simulink model "imu"  (R2015a)
settings: Solver=FixedStepDiscrete  StartTime=0.0  StopTime=inf  FixedStep=sample_time  RelTol=1e-3
values from neighbouring files (symbols this model uses):
  sample_time = 0.001    [ElmoIncremental.m]    (also in MedullaEncoder.m)
undefined symbols (not defined in the file or in its folder): imu_heading, imu_latitude, imu_reset_cmd
settings Model: xpc_rtwmakecfg_data=_xpcethercatlib_  SimulationMode=external  CovSFcnEnable=off  Creator=wmartin  LastModifiedBy=drl
settings SolverCC: EnableConcurrentExecution=on
settings DataIOCC: MaxDataPoints=1000000000  SaveFormat=StructureWithTime  SaveOutput=off  SaveTime=off
settings OptimizationCC: BlockReduction=off  OptimizeBlockIOStorage=off  BufferReuse=off  GlobalBufferReuse=off  ExpressionFolding=off  ExpressionDepthLimit=2147483647  LocalBlockOutputs=off  SimCompilerOptimization=on
settings DebuggingCC: ArtificialAlgebraicLoopMsg=none  UnderspecifiedInitializationDetection=Classic  MergeDetectMultiDrivingBlocksExec=none  SolverPrmCheckMsg=warning  StateNameClashWarn=warning
settings HardwareCC: ProdIntDivRoundTo=Zero  ProdEndianess=LittleEndian  ProdLongLongMode=on  ProdHWDeviceType=Generic->32-bit x86 compatible
settings ModelReferenceCC: EnableParallelModelReferenceBuilds=on  ModelReferenceNumInstancesAllowed=Single  ModelReferenceMinAlgLoopOccurrences=on
settings RTWCC: SystemTargetFile=slrt.tlc  TemplateMakefile=slrt_default_tmf  Description=Simulink Real-Time  RTWVerbose=off  RTWCompilerOptimization=on
settings CodeAppCC: MaxIdLength=256
settings SimulinkRealTimeCC: GeneratePreprocessorConditionals=Disable all  RL32LogBufSizeModifier=100000000

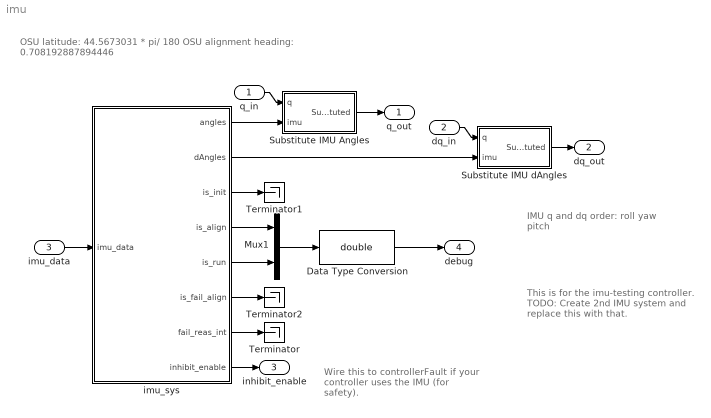
== system imu ==
  note: Wire this to controllerFault
      | if your controller uses the IMU
      | (for safety).
  note: This is for the imu-testing controller.
      | TODO: Create 2nd IMU system and
      | replace this with that.
  note: IMU q and dq order:
      | 	roll
      | 	yaw
      | 	pitch
  note: OSU latitude: 44.5673031 * pi/ 180
      | OSU alignment heading: 0.708192887894446
  q_in : Inport
  dq_in : Inport  Port=2
  imu_data : Inport  Port=3
  Data Type Conversion : DataTypeConversion  OutDataTypeStr=double
  Mux1 : Mux  Inputs=2
  Substitute IMU Angles : Subsystem
  Substitute IMU dAngles : Subsystem
  Terminator : Terminator
  Terminator1 : Terminator
  Terminator2 : Terminator
  imu_sys : MATLAB Function  TreatAsAtomicUnit=on
  q_out : Outport
  dq_out : Outport  Port=2
  inhibit_enable : Outport  Port=3
  debug : Outport  Port=4
  wires:
  imu_data/1 -> imu_sys/1(imu_data)
  imu_sys/1(angles) -> Substitute IMU Angles/2(imu)
  imu_sys/2(dAngles) -> Substitute IMU dAngles/2(imu)
  imu_sys/8(inhibit_enable) -> inhibit_enable/1
  imu_sys/7(fail_reas_int) -> Terminator/1
  imu_sys/6(is_fail_align) -> Terminator2/1
  imu_sys/3(is_init) -> Terminator1/1
  imu_sys/4(is_align) -> Mux1/1
  imu_sys/5(is_run) -> Mux1/2
  Mux1/1 -> Data Type Conversion/1
  Data Type Conversion/1 -> debug/1
  q_in/1 -> Substitute IMU Angles/1(q)
  dq_in/1 -> Substitute IMU dAngles/1(q)
  Substitute IMU Angles/1(Substituted) -> q_out/1
  Substitute IMU dAngles/1(Substituted) -> dq_out/1

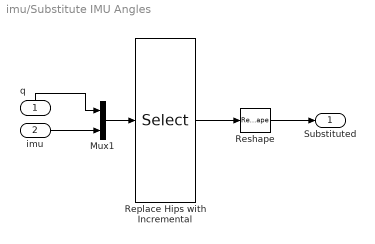
== system imu/Substitute IMU Angles ==
  q : Inport
  imu : Inport  Port=2
  Mux1 : Mux  Inputs=2
  Replace Hips with Incremental : Selector  InputPortWidth=16  Indices=[1 2 3 4 5 6 7 8 9 10 14 15 16]
  Reshape : Reshape
  Substituted : Outport
  wires:
  imu/1 -> Mux1/2
  q/1 -> Mux1/1
  Replace Hips with Incremental/1 -> Reshape/1
  Mux1/1 -> Replace Hips with Incremental/1
  Reshape/1 -> Substituted/1

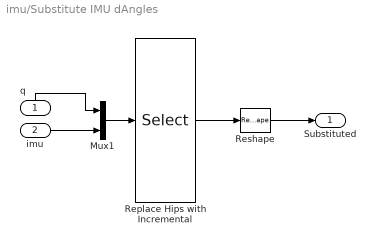
== system imu/Substitute IMU dAngles ==
  q : Inport
  imu : Inport  Port=2
  Mux1 : Mux  Inputs=2
  Replace Hips with Incremental : Selector  InputPortWidth=16  Indices=[1 2 3 4 5 6 7 8 9 10 14 15 16]
  Reshape : Reshape
  Substituted : Outport
  wires:
  Reshape/1 -> Substituted/1
  Mux1/1 -> Replace Hips with Incremental/1
  Replace Hips with Incremental/1 -> Reshape/1
  q/1 -> Mux1/1
  imu/1 -> Mux1/2

== matlab function imu/imu_sys ==
  data: imu_data input size=9; imu_latitude parameter size=1; imu_heading parameter size=1; angles output size=[3 1]; dAngles output size=[3 1]; sample_time parameter size=1; is_init output size=1; is_align output size=1; is_run output size=1; is_fail_align output size=1; fail_reas_int output size=1; inhibit_enable output size=1; imu_reset_cmd parameter
function [angles,dAngles,is_init,is_align,is_run,is_fail_align,fail_reas_int,inhibit_enable] ...
    = fcn(imu_data, imu_latitude, imu_heading, sample_time, imu_reset_cmd)
%#codegen

% State to trigger a reset only on the rising edge of imu_reset_cmd
persistent old_reset_cmd
if isempty(old_reset_cmd)
    old_reset_cmd = false;
end

% All our saved state is in these objects
persistent imusys coords

% Construct imusys at startup and whenever a reset is requested
if isempty(imusys) || (imu_reset_cmd && ~old_reset_cmd)
    imusys = imu.IMUSys(sample_time);
end

% Construct the coords object at startup
if isempty(coords)
    coords = imu.CmuCoords;
end

% Save old_reset_cmd for the next iteration
old_reset_cmd = logical(imu_reset_cmd);

% Run the IMU and BoomCoords objects
[local_orient, ang_vel, state, fail_reas] = ...
    imusys.update(imu_data(1:3), imu_data(4:6), uint8(imu_data(7)), uint8(imu_data(8)), imu_latitude, imu_heading);

[roll, pitch, yaw, dRoll, dPitch, dYaw] = ...
    coords.update(local_orient, ang_vel);

% Fully define our outputs to make MATLAB happy
angles  = [roll;  yaw;  pitch ];
dAngles = [dRoll; dYaw; dPitch];

% Create some additional diagnostic outputs
is_init       = state == imu.IMUSysState.INIT;
is_align      = state == imu.IMUSysState.ALIGN;
is_run        = state == imu.IMUSysState.RUN;
is_fail_align = state == imu.IMUSysState.FAIL;

% This output can be fed into the estop safeties, and will prevent the
% robot from enabling when IMU data is not available.
inhibit_enable = state ~= imu.IMUSysState.RUN;

% Ewww Simulink...
% This works around a bug with data types
fail_reas_int = uint8(fail_reas);
